simulink model "pasp_16ip_16ch"  (Simulink 6.2)
settings: Solver=ode45  StartTime=0.0  StopTime=30000  RelTol=1e-3
undefined symbols (not defined in the file or in its folder): iBOB
libraries: xbsIndex_r3 x1479, casper_library x149, xps_library x58
(part 2 of 11)

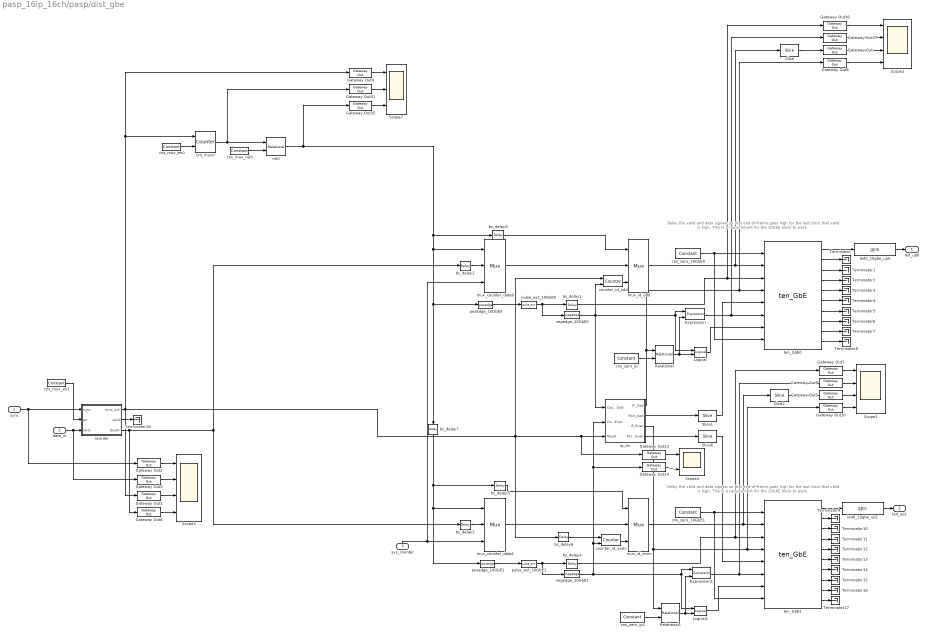
== system pasp_16ip_16ch/pasp/dist_gbe ==
  note: Delay the valid and data signals so that
      | end-of-frame goes high for the last clock
      | that valid is high. This is a requirement for
      | the 10GbE block to work.
  note: Delay the valid and data signals so that
      | end-of-frame goes high for the last clock
      | that valid is high. This is a requirement for
      | the 10GbE block to work.
  sync : Inport  Port=1  LatchInput=off
  data_in : Inport  Port=2  LatchInput=off
  sys_counter : Inport  Orientation=up  Port=3  LatchInput=off
  Expression : xbsIndex_r3/Expression  expression=a & ~b  precision=Full  arith_type=Unsigned  n_bits=8  bin_pt=2  align_bp=on  latency=0  explicit_period=off  period=1  en=off  dbl_ovrd=off  show_param=off
      settings: xl_area=[0, 0, 0, 0, 0, 0, 0]
  Expression1 : xbsIndex_r3/Expression  expression=a & ~b  precision=Full  arith_type=Unsigned  n_bits=8  bin_pt=2  align_bp=on  latency=0  explicit_period=off  period=1  en=off  dbl_ovrd=off  show_param=off
      settings: xl_area=[0, 0, 0, 0, 0, 0, 0]
  Gateway Out{,1..10,13..14,31,35..37} (17 alike) : xbsIndex_r3/Gateway Out  output_type=Double  nbits=8  bin_pt=6  arith_type=Boolean  quantization=Truncate  overflow=Wrap  hdl_port=on  timing_constraint=None  locs_specified=off  LOCs={}  needs_fixed_name=off  show_param=off
      settings: xl_area=[0, 0, 0, 0, 0, 0, 0]
  Logical : xbsIndex_r3/Logical  logical_function=AND  inputs=2  precision=Full  arith_type=Unsigned  n_bits=8  bin_pt=2  align_bp=on  latency=0  explicit_period=off  period=1  en=off  dbl_ovrd=off  show_param=off
      settings: xl_area=[0, 0, 0, 0, 0, 0, 0]
  Logical1 : xbsIndex_r3/Logical  logical_function=AND  inputs=2  precision=Full  arith_type=Unsigned  n_bits=8  bin_pt=2  align_bp=on  latency=0  explicit_period=off  period=1  en=off  dbl_ovrd=off  show_param=off
      settings: xl_area=[0, 0, 0, 0, 0, 0, 0]
  Relational : xbsIndex_r3/Relational  mode=a=b  latency=1  explicit_period=off  period=1  en=off  dbl_ovrd=off  show_param=off
      settings: xl_area=[0, 0, 0, 0, 0, 0, 0]
  Relational1 : xbsIndex_r3/Relational  mode=a=b  latency=1  explicit_period=off  period=1  en=off  dbl_ovrd=off  show_param=off
      settings: xl_area=[0, 0, 0, 0, 0, 0, 0]
  Scope1 : Scope  NumInputPorts=4
      settings: TimeRange=10000  YMin=0~0~0~4000  YMax=1~1~16~4016
  Scope2 : Scope  NumInputPorts=4
      settings: TimeRange=10000  YMin=0~0~0~0  YMax=1~1~10000~6.5e+010  SaveName=ScopeData2
  Scope3 : Scope  NumInputPorts=4
      settings: TimeRange=6000  YMin=0~0~-1~0  YMax=1~65~1~65  SaveName=ScopeData4
  Scope4 : Scope  NumInputPorts=2
      settings: TimeRange=10000  YMin=0~0  YMax=1~1  SaveName=ScopeData6
  Scope7 : Scope  NumInputPorts=3
      settings: YMin=0~0~0  YMax=1~275~1
  Slice : xbsIndex_r3/Slice  mode=Lower Bit Location + Width  nbits=5  bit1=0  base1=MSB of Input  bit0=0  base0=LSB of Input  boolean_output=off  explicit_period=off  period=1  dbl_ovrd=off
  Slice1 : xbsIndex_r3/Slice  mode=Lower Bit Location + Width  nbits=16  bit1=0  base1=MSB of Input  bit0=0  base0=LSB of Input  boolean_output=off  explicit_period=off  period=1  dbl_ovrd=off
  Slice2 : xbsIndex_r3/Slice  mode=Lower Bit Location + Width  nbits=5  bit1=0  base1=MSB of Input  bit0=0  base0=LSB of Input  boolean_output=off  explicit_period=off  period=1  dbl_ovrd=off
  Slice6 : xbsIndex_r3/Slice  mode=Lower Bit Location + Width  nbits=16  bit1=0  base1=MSB of Input  bit0=0  base0=LSB of Input  boolean_output=off  explicit_period=off  period=1  dbl_ovrd=off
  Terminator{,1..18} (19 alike) : Terminator
  bs_delay{1..2,4..5} (4 alike) : xbsIndex_r3/Delay  latency=1  reg_retiming=off  explicit_period=on  period=1  en=off  accept_only_valid=off  init_zero=on  dbl_ovrd=off  show_param=off
      settings: xl_area=[0, 0, 0, 0, 0, 0, 0]
  bs_delay3 : xbsIndex_r3/Delay  latency=2  reg_retiming=off  explicit_period=on  period=1  en=off  accept_only_valid=off  init_zero=on  dbl_ovrd=off  show_param=off
      settings: xl_area=[0, 0, 0, 0, 0, 0, 0]
  bs_delay6 : xbsIndex_r3/Delay  latency=4  reg_retiming=off  explicit_period=on  period=1  en=off  accept_only_valid=off  init_zero=on  dbl_ovrd=off  show_param=off
      settings: xl_area=[0, 0, 0, 0, 0, 0, 0]
  bs_delay7 : xbsIndex_r3/Delay  Orientation=down  latency=64  reg_retiming=off  explicit_period=on  period=1  en=off  accept_only_valid=off  init_zero=on  dbl_ovrd=off  show_param=off
      settings: xl_area=[0, 0, 0, 0, 0, 0, 0]
  bs_delay8 : xbsIndex_r3/Delay  latency=2  reg_retiming=off  explicit_period=on  period=1  en=off  accept_only_valid=off  init_zero=on  dbl_ovrd=off  show_param=off
      settings: xl_area=[0, 0, 0, 0, 0, 0, 0]
  cns_mux_en0 : xbsIndex_r3/Constant  const=1  equ=P=C  arith_type=Boolean  n_bits=1  bin_pt=0  opselect=C  inp2=PCIN>>17  opr=+  inp1=P  carry=CIN  iostate=0  explicit_period=on  period=1  dbl_ovrd=off
  cns_mux_en1 : xbsIndex_r3/Constant  const=1  equ=P=C  arith_type=Boolean  n_bits=1  bin_pt=0  opselect=C  inp2=PCIN>>17  opr=+  inp1=P  carry=CIN  iostate=0  explicit_period=on  period=1  dbl_ovrd=off
  cns_mux_rel0 : xbsIndex_r3/Constant  const=126  equ=P=C  arith_type=Unsigned  n_bits=7  bin_pt=0  opselect=C  inp2=PCIN>>17  opr=+  inp1=P  carry=CIN  iostate=0  explicit_period=on  period=1  dbl_ovrd=off
  cns_zero_10GbE0 : xbsIndex_r3/Constant  const=0  equ=P=C  arith_type=Boolean  n_bits=32  bin_pt=0  opselect=C  inp2=PCIN>>17  opr=+  inp1=P  carry=CIN  iostate=0  explicit_period=on  period=1  dbl_ovrd=off
  cns_zero_10GbE1 : xbsIndex_r3/Constant  const=0  equ=P=C  arith_type=Boolean  n_bits=32  bin_pt=0  opselect=C  inp2=PCIN>>17  opr=+  inp1=P  carry=CIN  iostate=0  explicit_period=on  period=1  dbl_ovrd=off
  cns_zero_ip : xbsIndex_r3/Constant  const=0  equ=P=C  arith_type=Unsigned  n_bits=32  bin_pt=0  opselect=C  inp2=PCIN>>17  opr=+  inp1=P  carry=CIN  iostate=0  explicit_period=on  period=1  dbl_ovrd=off
  cns_zero_ip1 : xbsIndex_r3/Constant  const=0  equ=P=C  arith_type=Unsigned  n_bits=32  bin_pt=0  opselect=C  inp2=PCIN>>17  opr=+  inp1=P  carry=CIN  iostate=0  explicit_period=on  period=1  dbl_ovrd=off
  cnt_mux0 : xbsIndex_r3/Counter  cnt_type=Free Running  n_bits=7  bin_pt=0  arith_type=Unsigned  start_count=0  cnt_to=Inf  cnt_by_val=1  operation=Up  explicit_period=off  period=1  load_pin=off  rst=on  en=on  dbl_ovrd=off  show_param=off  use_rpm=on  gen_core=off
      settings: xl_area=[0, 0, 0, 0, 0, 0, 0]
  counter_id_even : xbsIndex_r3/Counter  cnt_type=Count Limited  n_bits=64  bin_pt=0  arith_type=Unsigned  start_count=2  cnt_to=16  cnt_by_val=2  operation=Up  explicit_period=off  period=1  load_pin=off  rst=on  en=on  dbl_ovrd=off  show_param=off  use_rpm=on  gen_core=off
      settings: xl_area=[0, 0, 0, 0, 0, 0, 0]
  counter_id_odd : xbsIndex_r3/Counter  cnt_type=Count Limited  n_bits=64  bin_pt=0  arith_type=Unsigned  start_count=1  cnt_to=15  cnt_by_val=2  operation=Up  explicit_period=off  period=1  load_pin=off  rst=on  en=on  dbl_ovrd=off  show_param=off  use_rpm=on  gen_core=off
      settings: xl_area=[0, 0, 0, 0, 0, 0, 0]
  ip_ctr : Subsystem  mask(ip_ctr){numcomputers=16}
      mask prompts: numcomputers "Num IPs (Must be power of 2)"
      mask init:
      | ip_ctr_init(gcb,...
      |     'numcomputers',numcomputers)
      settings: AttributesFormatString=IPs=16
  led0_10gbe_up0 : xps_library/gpio  Tag=xps:gpio  io_group=iBOB:led  io_dir=out  arith_type=Boolean  bitwidth=1  bin_pt=0  bit_index=1  sample_period=1  use_single_ended=off  use_ddr=off  reg_iob=on  reg_clk_phase=0  termination=None
  led0_10gbe_up1 : xps_library/gpio  Tag=xps:gpio  io_group=iBOB:led  io_dir=out  arith_type=Boolean  bitwidth=1  bin_pt=0  bit_index=2  sample_period=1  use_single_ended=off  use_ddr=off  reg_iob=on  reg_clk_phase=0  termination=None
  mux_counter_data0 : xbsIndex_r3/Mux  inputs=2  precision=Full  arith_type="Signed  (2's comp)"  n_bits=8  bin_pt=2  quantization=Truncate  overflow=Wrap  latency=1  explicit_period=off  period=1  en=off  dbl_ovrd=off  show_param=off  mux_type=off  use_rpm=off  gen_core=off
      settings: xl_area=[0, 0, 0, 0, 0, 0, 0]
  mux_counter_data1 : xbsIndex_r3/Mux  inputs=2  precision=Full  arith_type="Signed  (2's comp)"  n_bits=8  bin_pt=2  quantization=Truncate  overflow=Wrap  latency=1  explicit_period=off  period=1  en=off  dbl_ovrd=off  show_param=off  mux_type=off  use_rpm=off  gen_core=off
      settings: xl_area=[0, 0, 0, 0, 0, 0, 0]
  mux_id_even : xbsIndex_r3/Mux  inputs=2  precision=Full  arith_type="Signed  (2's comp)"  n_bits=8  bin_pt=2  quantization=Truncate  overflow=Wrap  latency=1  explicit_period=off  period=1  en=off  dbl_ovrd=off  show_param=off  mux_type=off  use_rpm=off  gen_core=off
      settings: xl_area=[0, 0, 0, 0, 0, 0, 0]
  mux_id_odd : xbsIndex_r3/Mux  inputs=2  precision=Full  arith_type="Signed  (2's comp)"  n_bits=8  bin_pt=2  quantization=Truncate  overflow=Wrap  latency=1  explicit_period=off  period=1  en=off  dbl_ovrd=off  show_param=off  mux_type=off  use_rpm=off  gen_core=off
      settings: xl_area=[0, 0, 0, 0, 0, 0, 0]
  negedge_10GbE0 : casper_library/Misc/negedge  Tag=Rising Edge Detector
  negedge_10GbE1 : casper_library/Misc/negedge  Tag=Rising Edge Detector
  posedge_10GbE0 : casper_library/Misc/posedge  Tag=Rising Edge Detector
  posedge_10GbE1 : casper_library/Misc/posedge  Tag=Rising Edge Detector
  pulse_ext_10GbE0 : casper_library/Misc/pulse_ext  pulse_len=66
  pulse_ext_10GbE1 : casper_library/Misc/pulse_ext  pulse_len=66
  rel0 : xbsIndex_r3/Relational  mode=a=b  latency=1  explicit_period=off  period=1  en=off  dbl_ovrd=off  show_param=off
      settings: xl_area=[0, 0, 0, 0, 0, 0, 0]
  reorder : Subsystem  AncestorBlock=casper_library/Reorder/reorder  mask(reorder){map=[0 16 32 48 64 80 96 112 128 144 160 176 192 208 224 240 256 272 288 304 320 336 352 368 384 400 416 432 448 464 480 496 512 528 544 560 576 592 608 624 640 656 672 688 704 720 736 752 768 784 800 816 832 848 864 880 896 912 928 944 960 976 992 1008 1 17 33 49 65 81 97 113 129 145 161 177 193 209 225 241 257 273 289 305 321 337 353 369 385 401 417 433 449 465 481 497 513 529 545 561 577 593 609 625 641 657 673 689 705 721 737 753 769 785 801 817 833 849 865 881 897 913 929 945 961 977 993 1009 2 18 34 50 66 82 98 114 130 146 162 178 194 210 226 242 258 274 290 306 322 338 354 370 386 402 418 434 450 466 482 498 514 530 546 562 578 594 610 626 642 658 674 690 706 722 738 754 770 786 802 818 834 850 866 882 898 914 930 946 962 978 994 1010 3 19 35 51 67 83 99 115 131 147 163 179 195 211 227 243 259 275 291 307 323 339 355 371 387 403 419 435 451 467 483 499 515 531 547 563 579 595 611 627 643 659 675 691 707 723 739 755 771 787 803 819 835 851 867 883 899 915 931 947 963 979 995 1011 4 20 36 52 68 84 100 116 132 148 164 180 196 212 228 244 260 276 292 308 324 340 356 372 388 404 420 436 452 468 484 500 516 532 548 564 580 596 612 628 644 660 676 692 708 724 740 756 772 788 804 820 836 852 868 884 900 916 932 948 964 980 996 1012 5 21 37 53 69 85 101 117 133 149 165 181 197 213 229 245 261 277 293 309 325 341 357 373 389 405 421 437 453 469 485 501 517 533 549 565 581 597 613 629 645 661 677 693 709 725 741 757 773 789 805 821 837 853 869 885 901 917 933 949 965 981 997 1013 6 22 38 54 70 86 102 118 134 150 166 182 198 214 230 246 262 278 294 310 326 342 358 374 390 406 422 438 454 470 486 502 518 534 550 566 582 598 614 630 646 662 678 694 710 726 742 758 774 790 806 822 838 854 870 886 902 918 934 950 966 982 998 1014 7 23 39 55 71 87 103 119 135 151 167 183 199 215 231 247 263 279 295 311 327 343 359 375 391 407 423 439 455 471 487 503 519 535 551 567 583 599 615 631 647 663 679 695 711 727 743 759 775 791 807 823 839 855 871 887 903 919 935 951 967 983 999 1015 8 24 40 56 72 88 104 120 136 152 168 184 200 216 232 248 264 280 296 312 328 344 360 376 392 408 424 440 456 472 488 504 520 536 552 568 584 600 616 632 648 664 680 696 712 728 744 760 776 792 808 824 840 856 872 888 904 920 936 952 968 984 1000 1016 9 25 41 57 73 89 105 121 137 153 169 185 201 217 233 249 265 281 297 313 329 345 361 377 393 409 425 441 457 473 489 505 521 537 553 569 585 601 617 633 649 665 681 697 713 729 745 761 777 793 809 825 841 857 873 889 905 921 937 953 969 985 1001 1017 10 26 42 58 74 90 106 122 138 154 170 186 202 218 234 250 266 282 298 314 330 346 362 378 394 410 426 442 458 474 490 506 522 538 554 570 586 602 618 634 650 666 682 698 714 730 746 762 778 794 810 826 842 858 874 890 906 922 938 954 970 986 1002 1018 11 27 43 59 75 91 107 123 139 155 171 187 203 219 235 251 267 283 299 315 331 347 363 379 395 411 427 443 459 475 491 507 523 539 555 571 587 603 619 635 651 667 683 699 715 731 747 763 779 795 811 827 843 859 875 891 907 923 939 955 971 987 1003 1019 12 28 44 60 76 92 108 124 140 156 172 188 204 220 236 252 268 284 300 316 332 348 364 380 396 412 428 444 460 476 492 508 524 540 556 572 588 604 620 636 652 668 684 700 716 732 748 764 780 796 812 828 844 860 876 892 908 924 940 956 972 988 1004 1020 13 29 45 61 77 93 109 125 141 157 173 189 205 221 237 253 269 285 301 317 333 349 365 381 397 413 429 445 461 477 493 509 525 541 557 573 589 605 621 637 653 669 685 701 717 733 749 765 781 797 813 829 845 861 877 893 909 925 941 957 973 989 1005 1021 14 30 46 62 78 94 110 126 142 158 174 190 206 222 238 254 270 286 302 318 334 350 366 382 398 414 430 446 462 478 494 510 526 542 558 574 590 606 622 638 654 670 686 702 718 734 750 766 782 798 814 830 846 862 878 894 910 926 942 958 974 990 1006 1022 15 31 47 63 79 95 111 127 143 159 175 191 207 223 239 255 271 287 303 319 335 351 367 383 399 415 431 447 463 479 495 511 527 543 559 575 591 607 623 639 655 671 687 703 719 735 751 767 783 799 815 831 847 863 879 895 911 927 943 959 975 991 1007 1023], n_inputs=1, bram_latency=2, map_latency=1, double_buffer=1}
      mask prompts: map "Output Order:"; n_inputs "Number of inputs"; bram_latency "BRAM Latency"; map_latency "Map Latency"; double_buffer "Double Buffer"
      mask init:
      | reorder_init(gcb, ...
      |     'map', map, ...
      |     'n_inputs', n_inputs, ...
      |     'bram_latency', bram_latency, ...
      |     'map_latency', map_latency, ...
      |     'double_buffer', double_buffer);
      settings: AttributesFormatString=order=2
  ten_GbE0 : xps_library/ten_GbE  Tag=xps:tengbe  port=iBOB:0  mac_lite=on  show_param=on  pre_emph=2  swing=800
  ten_GbE1 : xps_library/ten_GbE  Tag=xps:tengbe  port=iBOB:1  mac_lite=on  show_param=on  pre_emph=2  swing=800
  led_up0 : Outport
  led_up1 : Outport  Port=2
  wires:
  sys_counter/1 -> mux_counter_data1/3, mux_counter_data0/3
  data_in/1 -> Gateway Out3/1, reorder/3(din0)
  reorder/2(valid) -> Terminator18/1
  Gateway Out36/1 -> Scope1/1
  ten_GbE1/10 -> Terminator17/1
  ten_GbE1/9 -> Terminator16/1
  ten_GbE1/8 -> Terminator15/1
  ten_GbE1/7 -> Terminator14/1
  ten_GbE1/6 -> Terminator13/1
  ten_GbE1/5 -> Terminator12/1
  ten_GbE1/4 -> Terminator11/1
  ten_GbE1/3 -> Terminator10/1
  ten_GbE1/2 -> Terminator9/1
  ten_GbE0/10 -> Terminator8/1
  ten_GbE0/9 -> Terminator7/1
  ten_GbE0/8 -> Terminator6/1
  ten_GbE0/7 -> Terminator5/1
  ten_GbE0/6 -> Terminator4/1
  ten_GbE0/5 -> Terminator3/1
  ten_GbE0/4 -> Terminator2/1
  ten_GbE0/3 -> Terminator1/1
  ten_GbE0/2 -> Terminator/1
  ten_GbE0/1 -> led0_10gbe_up0/1
  cns_zero_10GbE0/1 -> ten_GbE0/1, ten_GbE0/8
  mux_counter_data0/1 -> mux_id_odd/2
  cnt_mux0/1 -> rel0/1, Gateway Out31/1
  cns_mux_en0/1 -> cnt_mux0/2
  Gateway Out37/1 -> Scope1/2
  Gateway Out/1 -> Scope1/3
  pulse_ext_10GbE0/1 -> bs_delay1/1, negedge_10GbE0/1
  negedge_10GbE0/1 -> Logical/1, Expression/1, ip_ctr/1(Count_Odd), counter_id_odd/2
  cns_mux_rel0/1 -> rel0/2
  rel0/1 -> Gateway Out35/1, mux_counter_data0/1, posedge_10GbE0/1, bs_delay7/1, bs_delay8/1
  posedge_10GbE0/1 -> pulse_ext_10GbE0/1
  bs_delay1/1 -> ten_GbE0/3, Gateway Out36/1
  mux_id_odd/1 -> ten_GbE0/2, Slice/1
  Gateway Out4/1 -> Scope7/1
  Gateway Out31/1 -> Scope7/2
  Gateway Out35/1 -> Scope7/3
  bs_delay2/1 -> mux_counter_data0/2
  ten_GbE1/1 -> led0_10gbe_up1/1
  cns_zero_10GbE1/1 -> ten_GbE1/1, ten_GbE1/8
  mux_counter_data1/1 -> mux_id_even/2
  pulse_ext_10GbE1/1 -> negedge_10GbE1/1, bs_delay4/1
  negedge_10GbE1/1 -> Logical1/1, Expression1/1, counter_id_even/2, ip_ctr/2(Count_Even), Gateway Out14/1
  posedge_10GbE1/1 -> pulse_ext_10GbE1/1
  bs_delay4/1 -> ten_GbE1/3, Gateway Out7/1
  mux_id_even/1 -> ten_GbE1/2, Slice2/1
  bs_delay5/1 -> mux_counter_data1/2
  bs_delay7/1 -> mux_counter_data1/1, posedge_10GbE1/1, bs_delay3/1
  Gateway Out9/1 -> Scope2/2
  reorder/3(dout0) -> bs_delay5/1, bs_delay2/1, Gateway Out6/1
  cns_mux_en1/1 -> reorder/2(en)
  Gateway Out2/1 -> Scope3/1
  Gateway Out3/1 -> Scope3/2
  Gateway Out1/1 -> Scope3/3
  Gateway Out6/1 -> Scope3/4
  reorder/1(sync_out) -> Gateway Out1/1, cnt_mux0/1, Gateway Out4/1, counter_id_odd/1, ip_ctr/3(Reset), Gateway Out13/1, bs_delay6/1
  sync/1 -> reorder/1(sync), Gateway Out2/1
  led0_10gbe_up0/1 -> led_up0/1
  led0_10gbe_up1/1 -> led_up1/1
  cns_zero_ip/1 -> Relational/2
  Logical/1 -> ten_GbE0/7
  Relational/1 -> Logical/2, Expression/2
  Expression/1 -> ten_GbE0/6, Gateway Out37/1
  Relational1/1 -> Logical1/2, Expression1/2
  Logical1/1 -> ten_GbE1/7
  Expression1/1 -> ten_GbE1/6, Gateway Out9/1
  cns_zero_ip1/1 -> Relational1/2
  Gateway Out8/1 -> Scope1/4
  Slice/1 -> Gateway Out/1
  ip_ctr/2(Port_Odd) -> Slice1/1
  Slice1/1 -> ten_GbE0/5
  Slice6/1 -> ten_GbE1/5
  Slice2/1 -> Gateway Out5/1
  ip_ctr/4(Port_Even) -> Slice6/1
  ip_ctr/1(IP_Odd) -> Relational/1, ten_GbE0/4, Gateway Out8/1
  Gateway Out7/1 -> Scope2/1
  Gateway Out5/1 -> Scope2/3
  Gateway Out10/1 -> Scope2/4
  bs_delay8/1 -> mux_id_odd/1
  counter_id_odd/1 -> mux_id_odd/3
  bs_delay3/1 -> mux_id_even/1
  counter_id_even/1 -> mux_id_even/3
  Gateway Out14/1 -> Scope4/2
  Gateway Out13/1 -> Scope4/1
  ip_ctr/3(IP_Even) -> Relational1/1, ten_GbE1/4, Gateway Out10/1
  bs_delay6/1 -> counter_id_even/1

== system pasp_16ip_16ch/pasp/fft_wideband_real ==
  sync : Inport  Port=1  LatchInput=off
  shift : Inport  Port=2  LatchInput=off
  in0 : Inport  Port=3  LatchInput=off
  in1 : Inport  Port=4  LatchInput=off
  in2 : Inport  Port=5  LatchInput=off
  in3 : Inport  Port=6  LatchInput=off
  fft_biplex_real_4x0 : Subsystem  AncestorBlock=casper_library/FFTs/fft_biplex_real_4x  mask(fft_biplex_real_4x){FFTSize=3, BitWidth=18, quantization=Truncate, overflow=Wrap, add_latency=2, mult_latency=3, bram_latency=2}
      mask prompts: FFTSize "Size of FFT: (2^? pnts)"; BitWidth "Bitwidth: (Max Efficiency at 18 bits)"; quantization "Quantization Behavior"; overflow "Overflow Behavior"; add_latency "Add Latency"; mult_latency "Mult Latency"; bram_latency "BRAM Latency"
      mask init:
      | fft_biplex_real_4x_init(gcb,...
      |     'FFTSize', FFTSize,...
      |     'BitWidth', BitWidth,...
      |     'quantization', quantization,...
      |     'overflow', overflow,...
      |     'add_latency', add_latency,...
      |     'mult_latency', mult_latency,...
      |     'bram_latency', bram_latency);
      settings: AttributesFormatString=FFTSize=3, BitWidth=18
      mask StyleString: edit,edit,popup(Truncate|Round  (unbiased: +/- Inf)|Round  (unbiased: Even Values)),popup(Wrap|Saturate|Error),edit,edit,edit
  fft_direct : Subsystem  AncestorBlock=casper_library/FFTs/fft_direct  mask(fft_direct){FFTSize=2, BitWidth=18, add_latency=2, mult_latency=3, bram_latency=2, quantization=Truncate, overflow=Wrap, MapTail=1, LargerFFTSize=5, StartStage=4}
      mask prompts: FFTSize "Size of FFT: (2^?)"; BitWidth "Bit Width"; add_latency "Add Latency"; mult_latency "Mult Latency"; bram_latency "BRAM Latency"; quantization "Quantization Behavior"; overflow "Overflow Behavior"; MapTail "Map Tail of Larger FFT"; LargerFFTSize "Size of Larger FFT (2^?):"; StartStage "Start Stage of Map Tail:"
      mask init:
      | fft_direct_init(gcb,...
      |     'FFTSize', FFTSize,...
      |     'BitWidth', BitWidth,...
      |     'add_latency', add_latency,...
      |     'mult_latency', mult_latency,...
      |     'bram_latency', bram_latency,...
      |     'quantization', quantization,...
      |     'overflow', overflow,...
      |     'MapTail', MapTail,...
      |     'LargerFFTSize', LargerFFTSize,...
      |     'StartStage', StartStage);
      settings: AttributesFormatString=FFTSize=2
      mask StyleString: edit,edit,edit,edit,edit,popup(Truncate|Round  (unbiased: +/- Inf)|Round  (unbiased: Even Values)),popup(Wrap|Saturate|Error),edit,edit,edit
  fft_unscrambler : Subsystem  AncestorBlock=casper_library/FFTs/fft_unscrambler  mask(fft_unscrambler){FFTSize=4, n_inputs=1, bram_latency=2}
      mask prompts: FFTSize "Size of FFT: (2^?)"; n_inputs "Number of Simultaneous Inputs: (2^?)"; bram_latency "BRAM Latency"
      mask init:
      | fft_unscrambler_init(gcb,...
      |     'FFTSize',FFTSize,... 
      |     'n_inputs', n_inputs,...
      |     'bram_latency', bram_latency);
      settings: AttributesFormatString=FFTSize=4, n_inputs=1
  slice : xbsIndex_r3/Slice  mode=Lower Bit Location + Width  nbits=2  bit1=0  base1=MSB of Input  bit0=3  base0=LSB of Input  boolean_output=off  explicit_period=off  period=1  dbl_ovrd=off
  sync_out : Outport
  out0 : Outport  Port=2
  out1 : Outport  Port=3
  wires:
  in0/1 -> fft_biplex_real_4x0/1(pol1)
  in1/1 -> fft_biplex_real_4x0/2(pol2)
  in2/1 -> fft_biplex_real_4x0/3(pol3)
  in3/1 -> fft_biplex_real_4x0/4(pol4)
  shift/1 -> fft_biplex_real_4x0/6(shift), slice/1
  sync/1 -> fft_biplex_real_4x0/5(sync)
  slice/1 -> fft_direct/2(shift)
  fft_biplex_real_4x0/6(sync_out) -> fft_direct/1(sync)
  fft_biplex_real_4x0/1(pol1_out) -> fft_direct/3(in0)
  fft_biplex_real_4x0/2(pol2_out) -> fft_direct/4(in1)
  fft_biplex_real_4x0/3(pol3_out) -> fft_direct/5(in2)
  fft_biplex_real_4x0/4(pol4_out) -> fft_direct/6(in3)
  fft_direct/1(sync_out) -> fft_unscrambler/1(sync)
  fft_unscrambler/1(sync_out) -> sync_out/1
  fft_direct/2(out0) -> fft_unscrambler/2(In1)
  fft_unscrambler/2(Out1) -> out0/1
  fft_direct/3(out1) -> fft_unscrambler/3(In2)
  fft_unscrambler/3(Out2) -> out1/1

== system pasp_16ip_16ch/pasp/fft_wideband_real1 ==
  sync : Inport  Port=1  LatchInput=off
  shift : Inport  Port=2  LatchInput=off
  in0 : Inport  Port=3  LatchInput=off
  in1 : Inport  Port=4  LatchInput=off
  in2 : Inport  Port=5  LatchInput=off
  in3 : Inport  Port=6  LatchInput=off
  fft_biplex_real_4x0 : Subsystem  AncestorBlock=casper_library/FFTs/fft_biplex_real_4x  mask(fft_biplex_real_4x){FFTSize=3, BitWidth=18, quantization=Truncate, overflow=Wrap, add_latency=2, mult_latency=3, bram_latency=2}
      mask prompts: FFTSize "Size of FFT: (2^? pnts)"; BitWidth "Bitwidth: (Max Efficiency at 18 bits)"; quantization "Quantization Behavior"; overflow "Overflow Behavior"; add_latency "Add Latency"; mult_latency "Mult Latency"; bram_latency "BRAM Latency"
      mask init: same as pasp_16ip_16ch/pasp/fft_wideband_real/fft_biplex_real_4x0
      settings: AttributesFormatString=FFTSize=3, BitWidth=18
      mask StyleString: edit,edit,popup(Truncate|Round  (unbiased: +/- Inf)|Round  (unbiased: Even Values)),popup(Wrap|Saturate|Error),edit,edit,edit
  fft_direct : Subsystem  AncestorBlock=casper_library/FFTs/fft_direct  mask(fft_direct){FFTSize=2, BitWidth=18, add_latency=2, mult_latency=3, bram_latency=2, quantization=Truncate, overflow=Wrap, MapTail=1, LargerFFTSize=5, StartStage=4}
      mask prompts: FFTSize "Size of FFT: (2^?)"; BitWidth "Bit Width"; add_latency "Add Latency"; mult_latency "Mult Latency"; bram_latency "BRAM Latency"; quantization "Quantization Behavior"; overflow "Overflow Behavior"; MapTail "Map Tail of Larger FFT"; LargerFFTSize "Size of Larger FFT (2^?):"; StartStage "Start Stage of Map Tail:"
      mask init: same as pasp_16ip_16ch/pasp/fft_wideband_real/fft_direct
      settings: AttributesFormatString=FFTSize=2
      mask StyleString: edit,edit,edit,edit,edit,popup(Truncate|Round  (unbiased: +/- Inf)|Round  (unbiased: Even Values)),popup(Wrap|Saturate|Error),edit,edit,edit
  fft_unscrambler : Subsystem  AncestorBlock=casper_library/FFTs/fft_unscrambler  mask(fft_unscrambler){FFTSize=4, n_inputs=1, bram_latency=2}
      mask prompts: FFTSize "Size of FFT: (2^?)"; n_inputs "Number of Simultaneous Inputs: (2^?)"; bram_latency "BRAM Latency"
      mask init:
      | fft_unscrambler_init(gcb,...
      |     'FFTSize',FFTSize,... 
      |     'n_inputs', n_inputs,...
      |     'bram_latency', bram_latency);
      settings: AttributesFormatString=FFTSize=4, n_inputs=1
  slice : xbsIndex_r3/Slice  mode=Lower Bit Location + Width  nbits=2  bit1=0  base1=MSB of Input  bit0=3  base0=LSB of Input  boolean_output=off  explicit_period=off  period=1  dbl_ovrd=off
  sync_out : Outport
  out0 : Outport  Port=2
  out1 : Outport  Port=3
  wires:
  in0/1 -> fft_biplex_real_4x0/1(pol1)
  in1/1 -> fft_biplex_real_4x0/2(pol2)
  in2/1 -> fft_biplex_real_4x0/3(pol3)
  in3/1 -> fft_biplex_real_4x0/4(pol4)
  shift/1 -> fft_biplex_real_4x0/6(shift), slice/1
  sync/1 -> fft_biplex_real_4x0/5(sync)
  slice/1 -> fft_direct/2(shift)
  fft_biplex_real_4x0/6(sync_out) -> fft_direct/1(sync)
  fft_biplex_real_4x0/1(pol1_out) -> fft_direct/3(in0)
  fft_biplex_real_4x0/2(pol2_out) -> fft_direct/4(in1)
  fft_biplex_real_4x0/3(pol3_out) -> fft_direct/5(in2)
  fft_biplex_real_4x0/4(pol4_out) -> fft_direct/6(in3)
  fft_direct/1(sync_out) -> fft_unscrambler/1(sync)
  fft_unscrambler/1(sync_out) -> sync_out/1
  fft_direct/2(out0) -> fft_unscrambler/2(In1)
  fft_unscrambler/2(Out1) -> out0/1
  fft_direct/3(out1) -> fft_unscrambler/3(In2)
  fft_unscrambler/3(Out2) -> out1/1

== system pasp_16ip_16ch/pasp/pfb_fir_real ==
  sync : Inport  Port=1  LatchInput=off
  pol1_in1 : Inport  Port=2  LatchInput=off
  pol1_in2 : Inport  Port=3  LatchInput=off
  pol1_in3 : Inport  Port=4  LatchInput=off
  pol1_in4 : Inport  Port=5  LatchInput=off
  pol1_in1_first_tap : Subsystem  AncestorBlock=casper_library/PFBs/first_tap_real  mask(first_tap_real){nput=0, PFBSize=5, CoeffBitWidth=8, TotalTaps=2, BitWidthIn=8, CoeffDistMem=1, CoeffRound=0, WindowType=hamming, mult_latency=2, bram_latency=2, n_inputs=2, fwidth=1}
      mask prompts: nput "This is input number:"; PFBSize "Size of PFB: (2^? pnts)"; CoeffBitWidth "Bitwidth of Coefficients:"; TotalTaps "Total Number of Taps:"; BitWidthIn "Input Bitwidth:"; CoeffDistMem "Implement Coeff Gen in Distributed Memory:"; CoeffRound "Round Coefficients?"; WindowType "Windowing Function:"; mult_latency "Mult Latency"; bram_latency "BRAM Latency"; n_inputs "Number of Simultaneous Inputs: (2^?)"; fwidth "Bit Width (normal=1)"
      mask init:
      | first_tap_real_init(gcb,...
      |     'nput', nput,...
      |     'PFBSize', PFBSize,...
      |     'CoeffBitWidth', CoeffBitWidth,...
      |     'TotalTaps', TotalTaps,...
      |     'BitWidthIn', BitWidthIn,...
      |     'CoeffDistMem', CoeffDistMem,...
      |     'CoeffRound', CoeffRound,...
      |     'WindowType', WindowType,...
      |     'mult_latency', mult_latency,...
      |     'bram_latency', bram_latency,...
      |     'n_inputs', n_inputs,...
      |     'fwidth', fwidth);
      settings: AttributesFormatString=input=0, taps=2
      mask StyleString: edit,edit,edit,edit,edit,edit,edit,popup(bartlett|barthannwin|blackman|blackmanharris|bohamwin|chebwin|flattopwin|gausswin|hamming|hann|kaiser|nuttallwin|parzenwin|rectwin|tukeywin|triang),edit,edit,edit,edit
  pol1_in1_last_tap : Subsystem  AncestorBlock=casper_library/PFBs/last_tap_real  mask(last_tap_real){TotalTaps=2, BitWidthIn=8, BitWidthOut=18, CoeffBitWidth=8, add_latency=1, mult_latency=2, quantization=Truncate}
      mask prompts: TotalTaps "Total Number of Taps:"; BitWidthIn "Input Bitwidth:"; BitWidthOut "Output Bitwidth:"; CoeffBitWidth "Coeff Bitwidth:"; add_latency "Add Latency"; mult_latency "Mult Latency"; quantization "Quantization Behavior"
      mask init:
      | last_tap_real_init(gcb,...
      |     'TotalTaps', TotalTaps,...
      |     'BitWidthIn', BitWidthIn,...
      |     'BitWidthOut', BitWidthOut,...
      |     'CoeffBitWidth', CoeffBitWidth,...
      |     'add_latency', add_latency,...
      |     'mult_latency', mult_latency,...
      |     'quantization', quantization);
      settings: AttributesFormatString=taps=2
      mask StyleString: edit,edit,edit,edit,edit,edit,popup(Truncate|Round  (unbiased: +/- Inf)|Round  (unbiased: Even Values))
  pol1_in2_first_tap : Subsystem  AncestorBlock=casper_library/PFBs/first_tap_real  mask(first_tap_real){nput=1, PFBSize=5, CoeffBitWidth=8, TotalTaps=2, BitWidthIn=8, CoeffDistMem=1, CoeffRound=0, WindowType=hamming, mult_latency=2, bram_latency=2, n_inputs=2, fwidth=1}
      mask prompts: nput "This is input number:"; PFBSize "Size of PFB: (2^? pnts)"; CoeffBitWidth "Bitwidth of Coefficients:"; TotalTaps "Total Number of Taps:"; BitWidthIn "Input Bitwidth:"; CoeffDistMem "Implement Coeff Gen in Distributed Memory:"; CoeffRound "Round Coefficients?"; WindowType "Windowing Function:"; mult_latency "Mult Latency"; bram_latency "BRAM Latency"; n_inputs "Number of Simultaneous Inputs: (2^?)"; fwidth "Bit Width (normal=1)"
      mask init: same as pasp_16ip_16ch/pasp/pfb_fir_real/pol1_in1_first_tap
      settings: AttributesFormatString=input=1, taps=2
      mask StyleString: edit,edit,edit,edit,edit,edit,edit,popup(bartlett|barthannwin|blackman|blackmanharris|bohamwin|chebwin|flattopwin|gausswin|hamming|hann|kaiser|nuttallwin|parzenwin|rectwin|tukeywin|triang),edit,edit,edit,edit
  pol1_in2_last_tap : Subsystem  AncestorBlock=casper_library/PFBs/last_tap_real  mask(last_tap_real){TotalTaps=2, BitWidthIn=8, BitWidthOut=18, CoeffBitWidth=8, add_latency=1, mult_latency=2, quantization=Truncate}
      mask prompts: TotalTaps "Total Number of Taps:"; BitWidthIn "Input Bitwidth:"; BitWidthOut "Output Bitwidth:"; CoeffBitWidth "Coeff Bitwidth:"; add_latency "Add Latency"; mult_latency "Mult Latency"; quantization "Quantization Behavior"
      mask init: same as pasp_16ip_16ch/pasp/pfb_fir_real/pol1_in1_last_tap
      settings: AttributesFormatString=taps=2
      mask StyleString: edit,edit,edit,edit,edit,edit,popup(Truncate|Round  (unbiased: +/- Inf)|Round  (unbiased: Even Values))
  pol1_in3_first_tap : Subsystem  AncestorBlock=casper_library/PFBs/first_tap_real  mask(first_tap_real){nput=2, PFBSize=5, CoeffBitWidth=8, TotalTaps=2, BitWidthIn=8, CoeffDistMem=1, CoeffRound=0, WindowType=hamming, mult_latency=2, bram_latency=2, n_inputs=2, fwidth=1}
      mask prompts: nput "This is input number:"; PFBSize "Size of PFB: (2^? pnts)"; CoeffBitWidth "Bitwidth of Coefficients:"; TotalTaps "Total Number of Taps:"; BitWidthIn "Input Bitwidth:"; CoeffDistMem "Implement Coeff Gen in Distributed Memory:"; CoeffRound "Round Coefficients?"; WindowType "Windowing Function:"; mult_latency "Mult Latency"; bram_latency "BRAM Latency"; n_inputs "Number of Simultaneous Inputs: (2^?)"; fwidth "Bit Width (normal=1)"
      mask init: same as pasp_16ip_16ch/pasp/pfb_fir_real/pol1_in1_first_tap
      settings: AttributesFormatString=input=2, taps=2
      mask StyleString: edit,edit,edit,edit,edit,edit,edit,popup(bartlett|barthannwin|blackman|blackmanharris|bohamwin|chebwin|flattopwin|gausswin|hamming|hann|kaiser|nuttallwin|parzenwin|rectwin|tukeywin|triang),edit,edit,edit,edit
  pol1_in3_last_tap : Subsystem  AncestorBlock=casper_library/PFBs/last_tap_real  mask(last_tap_real){TotalTaps=2, BitWidthIn=8, BitWidthOut=18, CoeffBitWidth=8, add_latency=1, mult_latency=2, quantization=Truncate}
      mask prompts: TotalTaps "Total Number of Taps:"; BitWidthIn "Input Bitwidth:"; BitWidthOut "Output Bitwidth:"; CoeffBitWidth "Coeff Bitwidth:"; add_latency "Add Latency"; mult_latency "Mult Latency"; quantization "Quantization Behavior"
      mask init: same as pasp_16ip_16ch/pasp/pfb_fir_real/pol1_in1_last_tap
      settings: AttributesFormatString=taps=2
      mask StyleString: edit,edit,edit,edit,edit,edit,popup(Truncate|Round  (unbiased: +/- Inf)|Round  (unbiased: Even Values))
  pol1_in4_first_tap : Subsystem  AncestorBlock=casper_library/PFBs/first_tap_real  mask(first_tap_real){nput=3, PFBSize=5, CoeffBitWidth=8, TotalTaps=2, BitWidthIn=8, CoeffDistMem=1, CoeffRound=0, WindowType=hamming, mult_latency=2, bram_latency=2, n_inputs=2, fwidth=1}
      mask prompts: nput "This is input number:"; PFBSize "Size of PFB: (2^? pnts)"; CoeffBitWidth "Bitwidth of Coefficients:"; TotalTaps "Total Number of Taps:"; BitWidthIn "Input Bitwidth:"; CoeffDistMem "Implement Coeff Gen in Distributed Memory:"; CoeffRound "Round Coefficients?"; WindowType "Windowing Function:"; mult_latency "Mult Latency"; bram_latency "BRAM Latency"; n_inputs "Number of Simultaneous Inputs: (2^?)"; fwidth "Bit Width (normal=1)"
      mask init: same as pasp_16ip_16ch/pasp/pfb_fir_real/pol1_in1_first_tap
      settings: AttributesFormatString=input=3, taps=2
      mask StyleString: edit,edit,edit,edit,edit,edit,edit,popup(bartlett|barthannwin|blackman|blackmanharris|bohamwin|chebwin|flattopwin|gausswin|hamming|hann|kaiser|nuttallwin|parzenwin|rectwin|tukeywin|triang),edit,edit,edit,edit
  pol1_in4_last_tap : Subsystem  AncestorBlock=casper_library/PFBs/last_tap_real  mask(last_tap_real){TotalTaps=2, BitWidthIn=8, BitWidthOut=18, CoeffBitWidth=8, add_latency=1, mult_latency=2, quantization=Truncate}
      mask prompts: TotalTaps "Total Number of Taps:"; BitWidthIn "Input Bitwidth:"; BitWidthOut "Output Bitwidth:"; CoeffBitWidth "Coeff Bitwidth:"; add_latency "Add Latency"; mult_latency "Mult Latency"; quantization "Quantization Behavior"
      mask init: same as pasp_16ip_16ch/pasp/pfb_fir_real/pol1_in1_last_tap
      settings: AttributesFormatString=taps=2
      mask StyleString: edit,edit,edit,edit,edit,edit,popup(Truncate|Round  (unbiased: +/- Inf)|Round  (unbiased: Even Values))
  sync_out : Outport
  pol1_out1 : Outport  Port=2
  pol1_out2 : Outport  Port=3
  pol1_out3 : Outport  Port=4
  pol1_out4 : Outport  Port=5
  wires:
  pol1_in1/1 -> pol1_in1_first_tap/1(din)
  sync/1 -> pol1_in1_first_tap/2(sync), pol1_in2_first_tap/2(sync), pol1_in3_first_tap/2(sync), pol1_in4_first_tap/2(sync)
  pol1_in1_first_tap/1(dout) -> pol1_in1_last_tap/1(din)
  pol1_in1_first_tap/2(sync_out) -> pol1_in1_last_tap/2(sync)
  pol1_in1_first_tap/3(coeff_out) -> pol1_in1_last_tap/3(coeff)
  pol1_in1_first_tap/4(taps_out) -> pol1_in1_last_tap/4(taps)
  pol1_in1_last_tap/1(dout) -> pol1_out1/1
  pol1_in1_last_tap/2(sync_out) -> sync_out/1
  pol1_in2/1 -> pol1_in2_first_tap/1(din)
  pol1_in2_first_tap/1(dout) -> pol1_in2_last_tap/1(din)
  pol1_in2_first_tap/2(sync_out) -> pol1_in2_last_tap/2(sync)
  pol1_in2_first_tap/3(coeff_out) -> pol1_in2_last_tap/3(coeff)
  pol1_in2_first_tap/4(taps_out) -> pol1_in2_last_tap/4(taps)
  pol1_in2_last_tap/1(dout) -> pol1_out2/1
  pol1_in3/1 -> pol1_in3_first_tap/1(din)
  pol1_in3_first_tap/1(dout) -> pol1_in3_last_tap/1(din)
  pol1_in3_first_tap/2(sync_out) -> pol1_in3_last_tap/2(sync)
  pol1_in3_first_tap/3(coeff_out) -> pol1_in3_last_tap/3(coeff)
  pol1_in3_first_tap/4(taps_out) -> pol1_in3_last_tap/4(taps)
  pol1_in3_last_tap/1(dout) -> pol1_out3/1
  pol1_in4/1 -> pol1_in4_first_tap/1(din)
  pol1_in4_first_tap/1(dout) -> pol1_in4_last_tap/1(din)
  pol1_in4_first_tap/2(sync_out) -> pol1_in4_last_tap/2(sync)
  pol1_in4_first_tap/3(coeff_out) -> pol1_in4_last_tap/3(coeff)
  pol1_in4_first_tap/4(taps_out) -> pol1_in4_last_tap/4(taps)
  pol1_in4_last_tap/1(dout) -> pol1_out4/1

== system pasp_16ip_16ch/pasp/pfb_fir_real1 ==
  sync : Inport  Port=1  LatchInput=off
  pol1_in1 : Inport  Port=2  LatchInput=off
  pol1_in2 : Inport  Port=3  LatchInput=off
  pol1_in3 : Inport  Port=4  LatchInput=off
  pol1_in4 : Inport  Port=5  LatchInput=off
  pol1_in1_first_tap : Subsystem  AncestorBlock=casper_library/PFBs/first_tap_real  mask(first_tap_real){nput=0, PFBSize=5, CoeffBitWidth=8, TotalTaps=3, BitWidthIn=8, CoeffDistMem=1, CoeffRound=0, WindowType=hamming, mult_latency=2, bram_latency=2, n_inputs=2, fwidth=1}
      mask prompts: nput "This is input number:"; PFBSize "Size of PFB: (2^? pnts)"; CoeffBitWidth "Bitwidth of Coefficients:"; TotalTaps "Total Number of Taps:"; BitWidthIn "Input Bitwidth:"; CoeffDistMem "Implement Coeff Gen in Distributed Memory:"; CoeffRound "Round Coefficients?"; WindowType "Windowing Function:"; mult_latency "Mult Latency"; bram_latency "BRAM Latency"; n_inputs "Number of Simultaneous Inputs: (2^?)"; fwidth "Bit Width (normal=1)"
      mask init: same as pasp_16ip_16ch/pasp/pfb_fir_real/pol1_in1_first_tap
      settings: AttributesFormatString=input=0, taps=3
      mask StyleString: edit,edit,edit,edit,edit,edit,edit,popup(bartlett|barthannwin|blackman|blackmanharris|bohamwin|chebwin|flattopwin|gausswin|hamming|hann|kaiser|nuttallwin|parzenwin|rectwin|tukeywin|triang),edit,edit,edit,edit
  pol1_in1_last_tap : Subsystem  AncestorBlock=casper_library/PFBs/last_tap_real  mask(last_tap_real){TotalTaps=3, BitWidthIn=8, BitWidthOut=18, CoeffBitWidth=8, add_latency=1, mult_latency=2, quantization=Truncate}
      mask prompts: TotalTaps "Total Number of Taps:"; BitWidthIn "Input Bitwidth:"; BitWidthOut "Output Bitwidth:"; CoeffBitWidth "Coeff Bitwidth:"; add_latency "Add Latency"; mult_latency "Mult Latency"; quantization "Quantization Behavior"
      mask init: same as pasp_16ip_16ch/pasp/pfb_fir_real/pol1_in1_last_tap
      settings: AttributesFormatString=taps=3
      mask StyleString: edit,edit,edit,edit,edit,edit,popup(Truncate|Round  (unbiased: +/- Inf)|Round  (unbiased: Even Values))
  pol1_in1_tap2 : casper_library/PFBs/tap_real
      link override delay/delay_bram/Constant2: equ=P=C
      link override sync_delay/Constant: equ=P=C
      link override sync_delay/Constant1: equ=P=C
      link override sync_delay/Constant2: equ=P=C
      link override sync_delay/Constant3: equ=P=C
  pol1_in2_first_tap : Subsystem  AncestorBlock=casper_library/PFBs/first_tap_real  mask(first_tap_real){nput=1, PFBSize=5, CoeffBitWidth=8, TotalTaps=3, BitWidthIn=8, CoeffDistMem=1, CoeffRound=0, WindowType=hamming, mult_latency=2, bram_latency=2, n_inputs=2, fwidth=1}
      mask prompts: nput "This is input number:"; PFBSize "Size of PFB: (2^? pnts)"; CoeffBitWidth "Bitwidth of Coefficients:"; TotalTaps "Total Number of Taps:"; BitWidthIn "Input Bitwidth:"; CoeffDistMem "Implement Coeff Gen in Distributed Memory:"; CoeffRound "Round Coefficients?"; WindowType "Windowing Function:"; mult_latency "Mult Latency"; bram_latency "BRAM Latency"; n_inputs "Number of Simultaneous Inputs: (2^?)"; fwidth "Bit Width (normal=1)"
      mask init: same as pasp_16ip_16ch/pasp/pfb_fir_real/pol1_in1_first_tap
      settings: AttributesFormatString=input=1, taps=3
      mask StyleString: edit,edit,edit,edit,edit,edit,edit,popup(bartlett|barthannwin|blackman|blackmanharris|bohamwin|chebwin|flattopwin|gausswin|hamming|hann|kaiser|nuttallwin|parzenwin|rectwin|tukeywin|triang),edit,edit,edit,edit
  pol1_in2_last_tap : Subsystem  AncestorBlock=casper_library/PFBs/last_tap_real  mask(last_tap_real){TotalTaps=3, BitWidthIn=8, BitWidthOut=18, CoeffBitWidth=8, add_latency=1, mult_latency=2, quantization=Truncate}
      mask prompts: TotalTaps "Total Number of Taps:"; BitWidthIn "Input Bitwidth:"; BitWidthOut "Output Bitwidth:"; CoeffBitWidth "Coeff Bitwidth:"; add_latency "Add Latency"; mult_latency "Mult Latency"; quantization "Quantization Behavior"
      mask init: same as pasp_16ip_16ch/pasp/pfb_fir_real/pol1_in1_last_tap
      settings: AttributesFormatString=taps=3
      mask StyleString: edit,edit,edit,edit,edit,edit,popup(Truncate|Round  (unbiased: +/- Inf)|Round  (unbiased: Even Values))
  pol1_in2_tap2 : casper_library/PFBs/tap_real
      link override delay/delay_bram/Constant2: equ=P=C
      link override sync_delay/Constant: equ=P=C
      link override sync_delay/Constant1: equ=P=C
      link override sync_delay/Constant2: equ=P=C
      link override sync_delay/Constant3: equ=P=C
  pol1_in3_first_tap : Subsystem  AncestorBlock=casper_library/PFBs/first_tap_real  mask(first_tap_real){nput=2, PFBSize=5, CoeffBitWidth=8, TotalTaps=3, BitWidthIn=8, CoeffDistMem=1, CoeffRound=0, WindowType=hamming, mult_latency=2, bram_latency=2, n_inputs=2, fwidth=1}
      mask prompts: nput "This is input number:"; PFBSize "Size of PFB: (2^? pnts)"; CoeffBitWidth "Bitwidth of Coefficients:"; TotalTaps "Total Number of Taps:"; BitWidthIn "Input Bitwidth:"; CoeffDistMem "Implement Coeff Gen in Distributed Memory:"; CoeffRound "Round Coefficients?"; WindowType "Windowing Function:"; mult_latency "Mult Latency"; bram_latency "BRAM Latency"; n_inputs "Number of Simultaneous Inputs: (2^?)"; fwidth "Bit Width (normal=1)"
      mask init: same as pasp_16ip_16ch/pasp/pfb_fir_real/pol1_in1_first_tap
      settings: AttributesFormatString=input=2, taps=3
      mask StyleString: edit,edit,edit,edit,edit,edit,edit,popup(bartlett|barthannwin|blackman|blackmanharris|bohamwin|chebwin|flattopwin|gausswin|hamming|hann|kaiser|nuttallwin|parzenwin|rectwin|tukeywin|triang),edit,edit,edit,edit
  pol1_in3_last_tap : Subsystem  AncestorBlock=casper_library/PFBs/last_tap_real  mask(last_tap_real){TotalTaps=3, BitWidthIn=8, BitWidthOut=18, CoeffBitWidth=8, add_latency=1, mult_latency=2, quantization=Truncate}
      mask prompts: TotalTaps "Total Number of Taps:"; BitWidthIn "Input Bitwidth:"; BitWidthOut "Output Bitwidth:"; CoeffBitWidth "Coeff Bitwidth:"; add_latency "Add Latency"; mult_latency "Mult Latency"; quantization "Quantization Behavior"
      mask init: same as pasp_16ip_16ch/pasp/pfb_fir_real/pol1_in1_last_tap
      settings: AttributesFormatString=taps=3
      mask StyleString: edit,edit,edit,edit,edit,edit,popup(Truncate|Round  (unbiased: +/- Inf)|Round  (unbiased: Even Values))
  pol1_in3_tap2 : casper_library/PFBs/tap_real
      link override delay/delay_bram/Constant2: equ=P=C
      link override sync_delay/Constant: equ=P=C
      link override sync_delay/Constant1: equ=P=C
      link override sync_delay/Constant2: equ=P=C
      link override sync_delay/Constant3: equ=P=C
  pol1_in4_first_tap : Subsystem  AncestorBlock=casper_library/PFBs/first_tap_real  mask(first_tap_real){nput=3, PFBSize=5, CoeffBitWidth=8, TotalTaps=3, BitWidthIn=8, CoeffDistMem=1, CoeffRound=0, WindowType=hamming, mult_latency=2, bram_latency=2, n_inputs=2, fwidth=1}
      mask prompts: nput "This is input number:"; PFBSize "Size of PFB: (2^? pnts)"; CoeffBitWidth "Bitwidth of Coefficients:"; TotalTaps "Total Number of Taps:"; BitWidthIn "Input Bitwidth:"; CoeffDistMem "Implement Coeff Gen in Distributed Memory:"; CoeffRound "Round Coefficients?"; WindowType "Windowing Function:"; mult_latency "Mult Latency"; bram_latency "BRAM Latency"; n_inputs "Number of Simultaneous Inputs: (2^?)"; fwidth "Bit Width (normal=1)"
      mask init: same as pasp_16ip_16ch/pasp/pfb_fir_real/pol1_in1_first_tap
      settings: AttributesFormatString=input=3, taps=3
      mask StyleString: edit,edit,edit,edit,edit,edit,edit,popup(bartlett|barthannwin|blackman|blackmanharris|bohamwin|chebwin|flattopwin|gausswin|hamming|hann|kaiser|nuttallwin|parzenwin|rectwin|tukeywin|triang),edit,edit,edit,edit
  pol1_in4_last_tap : Subsystem  AncestorBlock=casper_library/PFBs/last_tap_real  mask(last_tap_real){TotalTaps=3, BitWidthIn=8, BitWidthOut=18, CoeffBitWidth=8, add_latency=1, mult_latency=2, quantization=Truncate}
      mask prompts: TotalTaps "Total Number of Taps:"; BitWidthIn "Input Bitwidth:"; BitWidthOut "Output Bitwidth:"; CoeffBitWidth "Coeff Bitwidth:"; add_latency "Add Latency"; mult_latency "Mult Latency"; quantization "Quantization Behavior"
      mask init: same as pasp_16ip_16ch/pasp/pfb_fir_real/pol1_in1_last_tap
      settings: AttributesFormatString=taps=3
      mask StyleString: edit,edit,edit,edit,edit,edit,popup(Truncate|Round  (unbiased: +/- Inf)|Round  (unbiased: Even Values))
  pol1_in4_tap2 : casper_library/PFBs/tap_real
      link override delay/delay_bram/Constant2: equ=P=C
      link override sync_delay/Constant: equ=P=C
      link override sync_delay/Constant1: equ=P=C
      link override sync_delay/Constant2: equ=P=C
      link override sync_delay/Constant3: equ=P=C
  sync_out : Outport
  pol1_out1 : Outport  Port=2
  pol1_out2 : Outport  Port=3
  pol1_out3 : Outport  Port=4
  pol1_out4 : Outport  Port=5
  wires:
  pol1_in1/1 -> pol1_in1_first_tap/1(din)
  sync/1 -> pol1_in1_first_tap/2(sync), pol1_in2_first_tap/2(sync), pol1_in3_first_tap/2(sync), pol1_in4_first_tap/2(sync)
  pol1_in1_first_tap/1(dout) -> pol1_in1_tap2/1
  pol1_in1_first_tap/2(sync_out) -> pol1_in1_tap2/2
  pol1_in1_first_tap/3(coeff_out) -> pol1_in1_tap2/3
  pol1_in1_first_tap/4(taps_out) -> pol1_in1_tap2/4
  pol1_in1_tap2/1 -> pol1_in1_last_tap/1(din)
  pol1_in1_tap2/2 -> pol1_in1_last_tap/2(sync)
  pol1_in1_tap2/3 -> pol1_in1_last_tap/3(coeff)
  pol1_in1_tap2/4 -> pol1_in1_last_tap/4(taps)
  pol1_in1_last_tap/1(dout) -> pol1_out1/1
  pol1_in1_last_tap/2(sync_out) -> sync_out/1
  pol1_in2/1 -> pol1_in2_first_tap/1(din)
  pol1_in2_first_tap/1(dout) -> pol1_in2_tap2/1
  pol1_in2_first_tap/2(sync_out) -> pol1_in2_tap2/2
  pol1_in2_first_tap/3(coeff_out) -> pol1_in2_tap2/3
  pol1_in2_first_tap/4(taps_out) -> pol1_in2_tap2/4
  pol1_in2_tap2/1 -> pol1_in2_last_tap/1(din)
  pol1_in2_tap2/2 -> pol1_in2_last_tap/2(sync)
  pol1_in2_tap2/3 -> pol1_in2_last_tap/3(coeff)
  pol1_in2_tap2/4 -> pol1_in2_last_tap/4(taps)
  pol1_in2_last_tap/1(dout) -> pol1_out2/1
  pol1_in3/1 -> pol1_in3_first_tap/1(din)
  pol1_in3_first_tap/1(dout) -> pol1_in3_tap2/1
  pol1_in3_first_tap/2(sync_out) -> pol1_in3_tap2/2
  pol1_in3_first_tap/3(coeff_out) -> pol1_in3_tap2/3
  pol1_in3_first_tap/4(taps_out) -> pol1_in3_tap2/4
  pol1_in3_tap2/1 -> pol1_in3_last_tap/1(din)
  pol1_in3_tap2/2 -> pol1_in3_last_tap/2(sync)
  pol1_in3_tap2/3 -> pol1_in3_last_tap/3(coeff)
  pol1_in3_tap2/4 -> pol1_in3_last_tap/4(taps)
  pol1_in3_last_tap/1(dout) -> pol1_out3/1
  pol1_in4/1 -> pol1_in4_first_tap/1(din)
  pol1_in4_first_tap/1(dout) -> pol1_in4_tap2/1
  pol1_in4_first_tap/2(sync_out) -> pol1_in4_tap2/2
  pol1_in4_first_tap/3(coeff_out) -> pol1_in4_tap2/3
  pol1_in4_first_tap/4(taps_out) -> pol1_in4_tap2/4
  pol1_in4_tap2/1 -> pol1_in4_last_tap/1(din)
  pol1_in4_tap2/2 -> pol1_in4_last_tap/2(sync)
  pol1_in4_tap2/3 -> pol1_in4_last_tap/3(coeff)
  pol1_in4_tap2/4 -> pol1_in4_last_tap/4(taps)
  pol1_in4_last_tap/1(dout) -> pol1_out4/1
